simulink model "PID_Workshop"  (Simulink 9.3)
settings: Solver=ode4  StartTime=0.0  StopTime=inf  FixedStep=0.002  RelTol=1e-3  EnableMultiTasking=on
undefined symbols (not defined in the file): C, D, HIL, I, Kb, P, qc_get_step_size, Ref, V
libraries: quarc_library x6, simulink x1
settings Model: Creator=MLevis  LastModifiedBy=jxs210080  SimulationMode=external  ExtModeTrigDuration=1000000
settings SolverCC: PositivePriorityOrder=on
settings DataIOCC: LimitDataPoints=on
settings OptimizationCC: ExpressionDepthLimit=2147483647  InitFltsAndDblsToZero=on  LifeSpan=auto
settings DebuggingCC: SaveWithParameterizedLinksMsg=none  SolverPrmCheckMsg=warning  StateNameClashWarn=warning
settings SFSimCC: SimUseLocalCustomCode=on
settings RTWCC: SystemTargetFile=quarc_win64.tlc  TemplateMakefile=quarc_default_tmf  Description=QUARC Win64 Target  RTWUseLocalCustomCode=on
settings STFCustomTargetCC: TargetPreCompLibLocation=C:\PROGRA~3\QUARC\lib\2019a\win64\release  ConcurrentExecutionCompliant=on  SystemTargetFile=quarc_win64.tlc
settings GRTTargetCC: TargetPreCompLibLocation=C:\PROGRA~3\QUARC\lib\2019a\win64\release  ParMdlRefBuildCompliant=off  CompOptLevelCompliant=off  MatFileLogging=off  CPPClassGenCompliant=off  UseToolchainInfoCompliant=off  ExtMode=on  ExtModeMexFile=quarc_comm
settings ConfigComp: CovHtmlReporting=off  CovExternalEMLEnable=on

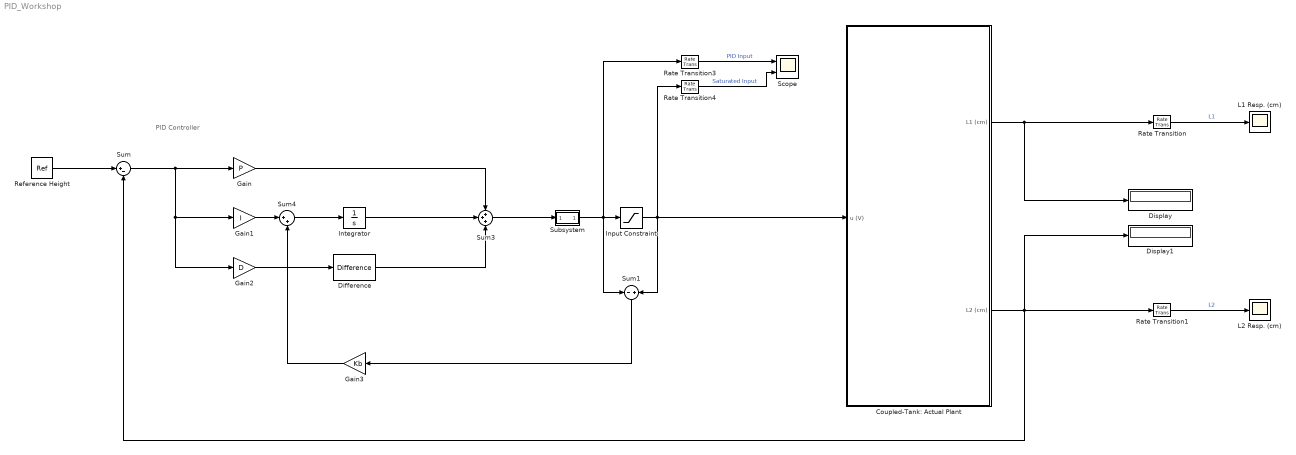
== system PID_Workshop ==
  note: PID Controller
  Coupled-Tank: Actual Plant : Subsystem
      mask Display: image('C:\Users\jxs210080\Downloads\Icon\two-tank system.png');
  Difference : simulink/Discrete/Difference  ICPrevInput=0.0  OutMin=[]  OutMax=[]  OutDataType=fixdt(1, 16)  OutScaling=2^-10  DoSatur=off
  Display : Display
  Display1 : Display
  Gain : Gain  Gain=P
  Gain1 : Gain  Gain=I
  Gain2 : Gain  Gain=D
  Gain3 : Gain  Gain=Kb
  Input Constraint : Saturate  UpperLimit=15  LowerLimit=0  LinearizeAsGain=off
  Integrator : Integrator  LimitOutput=on  UpperSaturationLimit=1000  LowerSaturationLimit=-1000
  L1 Resp. (cm) : Scope
  L2 Resp. (cm) : Scope
  Rate Transition{,1,3..4} (4 alike) : RateTransition  OutPortSampleTime=0.1
  Reference Height : Constant  Value=Ref
  Scope : Scope  NumInputPorts=2
  Subsystem : Subsystem
  Sum : Sum  Inputs=|+-
  Sum1 : Sum  Inputs=-|+
  Sum3 : Sum  Inputs=+++
  Sum4 : Sum  Inputs=|++
  wires:
  Coupled-Tank: Actual Plant/2(L2 (cm)) -> Display1/1, Rate Transition1/1, Sum/2
  Rate Transition/1 -> L1 Resp. (cm)/1  "L1"
  Rate Transition1/1 -> L2 Resp. (cm)/1  "L2"
  Sum/1 -> Gain2/1, Gain1/1, Gain/1
  Coupled-Tank: Actual Plant/1(L1 (cm)) -> Display/1, Rate Transition/1
  Reference Height/1 -> Sum/1
  Input Constraint/1 -> Coupled-Tank: Actual Plant/1(u (V)), Sum1/2, Rate Transition4/1
  Gain1/1 -> Sum4/1
  Gain2/1 -> Difference/1
  Integrator/1 -> Sum3/2
  Gain/1 -> Sum3/1
  Difference/1 -> Sum3/3
  Gain3/1 -> Sum4/2
  Sum4/1 -> Integrator/1
  Sum1/1 -> Gain3/1
  Subsystem/1(Out1) -> Input Constraint/1, Sum1/1, Rate Transition3/1
  Sum3/1 -> Subsystem/1(In1)
  Rate Transition3/1 -> Scope/1  "PID Input"
  Rate Transition4/1 -> Scope/2  "Saturated Input"

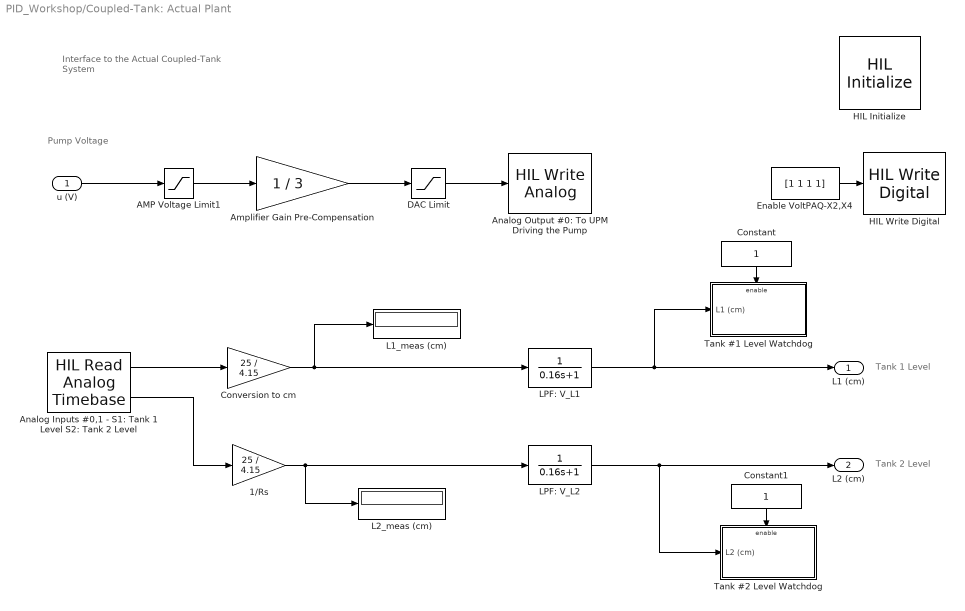
== system PID_Workshop/Coupled-Tank: Actual Plant ==
  note: Pump
      | Voltage
  note: Tank 2 Level
  note: Tank 1 Level
  note: Interface to the Actual
      | Coupled-Tank System
  u (V) : Inport
  1/Rs : Gain  Gain=25 / 4.15  SaturateOnIntegerOverflow=on  OutDataTypeStr=Inherit: Same as input  ParamDataTypeStr=Inherit: Same as input
  AMP Voltage Limit1 : Saturate  UpperLimit=22  LowerLimit=0
  Amplifier Gain Pre-Compensation : Gain  Gain=1 / 3  SaturateOnIntegerOverflow=on  OutDataTypeStr=Inherit: Same as input  ParamDataTypeStr=Inherit: Same as input
  Analog Inputs #0,1 - S1: Tank 1 Level S2: Tank 2 Level : quarc_library/Data Acquisition/Generic/Timebases/HIL Read Analog Timebase  object_name=HIL-2  clock=0  channels=[0:1]  samples_in_buffer=max(ceil(1/qc_get_step_size), 1)  active=on  vector_output=off
      settings: AttributesFormatString=(%<object_name>)  SourceProductName=QUARC Targets
  Analog Output #0: To UPM Driving the Pump : quarc_library/Data Acquisition/Generic/Immediate I//O/HIL Write Analog  object_name=HIL-2  channels=0  sample_time=-1  active=off  vector_input=off
  Constant : Constant
  Constant1 : Constant
  Conversion to cm : Gain  Gain=25 / 4.15  SaturateOnIntegerOverflow=on  OutDataTypeStr=Inherit: Same as input  ParamDataTypeStr=Inherit: Same as input
  DAC Limit : Saturate  UpperLimit=10  LowerLimit=-10
  Enable VoltPAQ-X2,X4 : Constant  Value=[1 1 1 1]
  HIL Initialize : quarc_library/Data Acquisition/Generic/Configuration/HIL Initialize  object_name=HIL-2  board_type=q2_usb  board_number=0  board_options=d0=digital;d1=digital;led=auto;update_rate=normal;decimation=1  exclusive=off  active=off  hardware_clocks=[0]  clock_modes=[]  initial_clock_frequencies=[]  set_clock_params_at_start=off  set_clock_params_at_switch_in=off  set_clock_frequencies_at_start=off  set_clock_frequencies_at_switch_in=off  analog_input_channels=[0:1]  analog_input_configurations=[]  analog_input_maximums=10  analog_input_minimums=-10  set_analog_input_params_at_start=on  set_analog_input_params_at_switch_in=off  analog_output_channels=[0:1]  analog_output_maximums=10  analog_output_minimums=-10  initial_analog_outputs=[0]  final_analog_outputs=[0]  watchdog_analog_outputs=0  set_analog_output_params_at_start=on  set_analog_output_params_at_switch_in=off  set_analog_outputs_at_start=on  set_analog_outputs_at_switch_in=off  set_analog_outputs_at_terminate=on  set_analog_outputs_at_switch_out=off  set_analog_outputs_on_watchdog=off  digital_input_channels=[]  digital_output_channels=[]  digital_output_configuration=[]  initial_digital_outputs=[1]  final_digital_outputs=[1]  watchdog_digital_outputs=[1]  set_digital_output_params_at_start=off  set_digital_output_params_at_switch_in=off  set_digital_outputs_at_start=on  set_digital_outputs_at_switch_in=off  set_digital_outputs_at_terminate=on  set_digital_outputs_at_switch_out=off  set_digital_outputs_on_watchdog=off  encoder_channels=[0:1]  quadrature=[4]  encoder_filter_frequency=[]  initial_encoder_counts=[0]  set_encoder_params_at_start=on  set_encoder_params_at_switch_in=off  set_encoder_counts_at_start=on  set_encoder_counts_at_switch_in=off  pwm_channels=[]  pwm_modes=[0]  pwm_frequency=1/0.020  pwm_configuration=[]  pwm_alignment=[]  pwm_polarity=[]  pwm_leading_deadband=[]  pwm_trailing_deadband=[]  initial_pwm_outputs=[0]  final_pwm_outputs=[0]  watchdog_pwm_outputs=[0]  set_pwm_params_at_start=on  set_pwm_params_at_switch_in=off  set_pwm_outputs_at_start=on  set_pwm_outputs_at_switch_in=off  set_pwm_outputs_at_terminate=on  set_pwm_outputs_at_switch_out=off  set_pwm_outputs_on_watchdog=off  other_output_channels=[]  initial_other_outputs=[]  final_other_outputs=[]  watchdog_other_outputs=[]  set_other_outputs_at_start=off  set_other_outputs_at_switch_in=off  set_other_outputs_at_terminate=off  set_other_outputs_at_switch_out=off  set_other_outputs_on_watchdog=off
  HIL Write Digital : quarc_library/Data Acquisition/Generic/Immediate I//O/HIL Write Digital  object_name=HIL-2  channels=[0:3]  sample_time=-1  active=off  vector_input=on
      settings: SourceProductName=QUARC Targets
  L1_meas (cm) : Display
      settings: Decimation=100
  L2_meas (cm) : Display
      settings: Decimation=100
  LPF: V_L1 : TransferFcn  Denominator=[0.16 1]
  LPF: V_L2 : TransferFcn  Denominator=[0.16 1]
  Tank #1 Level Watchdog : Subsystem  TreatAsAtomicUnit=on
  Tank #2 Level Watchdog : Subsystem  TreatAsAtomicUnit=on
  L1 (cm) : Outport  InitialOutput=0
  L2 (cm) : Outport  Port=2  InitialOutput=0
  wires:
  LPF: V_L2/1 -> Tank #2 Level Watchdog/1(L2 (cm)), L2 (cm)/1
  LPF: V_L1/1 -> Tank #1 Level Watchdog/1(L1 (cm)), L1 (cm)/1
  Constant1/1 -> Tank #2 Level Watchdog/Enable
  Constant/1 -> Tank #1 Level Watchdog/Enable
  Conversion to cm/1 -> LPF: V_L1/1, L1_meas (cm)/1
  DAC Limit/1 -> Analog Output #0: To UPM Driving the Pump/1
  1/Rs/1 -> LPF: V_L2/1, L2_meas (cm)/1
  Analog Inputs #0,1 - S1: Tank 1 Level S2: Tank 2 Level/2 -> 1/Rs/1
  Analog Inputs #0,1 - S1: Tank 1 Level S2: Tank 2 Level/1 -> Conversion to cm/1
  u (V)/1 -> AMP Voltage Limit1/1
  Amplifier Gain Pre-Compensation/1 -> DAC Limit/1
  Enable VoltPAQ-X2,X4/1 -> HIL Write Digital/1
  AMP Voltage Limit1/1 -> Amplifier Gain Pre-Compensation/1

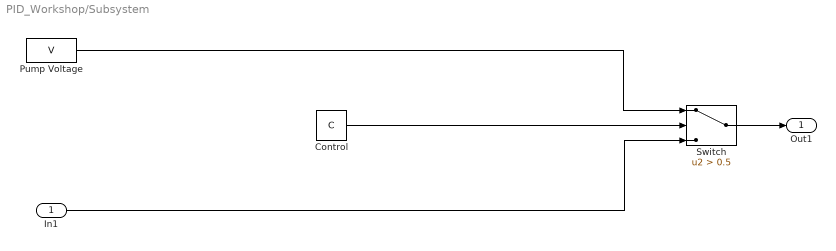
== system PID_Workshop/Subsystem ==
  In1 : Inport
  Control : Constant  Value=C
  Pump Voltage : Constant  Value=V
  Switch : Switch  Criteria=u2 > Threshold  Threshold=0.5
  Out1 : Outport  VectorParamsAs1DForOutWhenUnconnected=on
  wires:
  Pump Voltage/1 -> Switch/1
  Control/1 -> Switch/2
  In1/1 -> Switch/3
  Switch/1 -> Out1/1

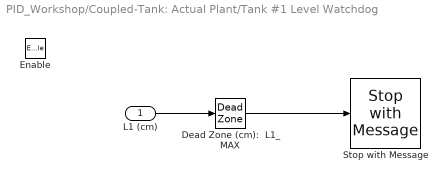
== system PID_Workshop/Coupled-Tank: Actual Plant/Tank #1 Level Watchdog ==
  L1 (cm) : Inport
  Enable : EnablePort
  Dead Zone (cm):  L1_MAX : DeadZone  LowerValue=-5  UpperValue=25  SaturateOnIntegerOverflow=on
  Stop with Message : quarc_library/Sinks/Error Handling/Stop with Message  message_type=Fixed error message  message_icon=Error  message=Tank #1 Level Limit Reached.
  wires:
  L1 (cm)/1 -> Dead Zone (cm):  L1_MAX/1
  Dead Zone (cm):  L1_MAX/1 -> Stop with Message/1

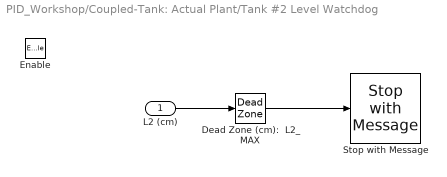
== system PID_Workshop/Coupled-Tank: Actual Plant/Tank #2 Level Watchdog ==
  L2 (cm) : Inport
  Enable : EnablePort
  Dead Zone (cm):  L2_MAX : DeadZone  LowerValue=-5  UpperValue=25  SaturateOnIntegerOverflow=on
  Stop with Message : quarc_library/Sinks/Error Handling/Stop with Message  message_type=Fixed error message  message_icon=Error  message=Tank #2 Level Limit Reached.
  wires:
  Dead Zone (cm):  L2_MAX/1 -> Stop with Message/1
  L2 (cm)/1 -> Dead Zone (cm):  L2_MAX/1
